simulink model "HANcoder_E407_Membership"  (R2022a)
settings: Solver=FixedStepDiscrete  StartTime=0.0  StopTime=1  FixedStep=0.01  RelTol=1e-3
PreLoadFcn:
  | librarySetup
  | eval([bdroot,'_startup']) %Calling [modelName]_startup.m
values from neighbouring files (symbols this model uses):
  HANtuneOverride = Simulink.Parameter    [HANcoder_E407_KinematicAngleControl_startup.m]    (also in HANcoder_E407_startup.m)
libraries: HANcoder_STM32_Target x14, simulink x2, simulink_extras x2, dspswit3 x1
settings Model: Creator=Jason van Kolfschoten  LastModifiedBy=luukr
settings SolverCC: AlgebraicLoopSolver=TrustRegion  PositivePriorityOrder=on
settings DataIOCC: LimitDataPoints=on  SaveFormat=Array  SignalLoggingSaveFormat=ModelDataLogs  SaveOutput=off  SignalLogging=off  DSMLogging=off  SaveTime=off  ReturnWorkspaceOutputs=off
settings OptimizationCC: BlockReduction=off  DefaultParameterBehavior=Inlined  DefaultUnderspecifiedDataType=single  InlineInvariantSignals=on  ExpressionDepthLimit=2147483647  StateBitsets=on  DataBitsets=on  ZeroExternalMemoryAtStartup=off  ZeroInternalMemoryAtStartup=off  InitFltsAndDblsToZero=on  NoFixptDivByZeroProtection=on  EfficientFloat2IntCast=on  LifeSpan=inf  EfficientTunableParamExpr=on
settings DebuggingCC: SaveWithDisabledLinksMsg=none  SaveWithParameterizedLinksMsg=none  CheckSSInitialOutputMsg=off  UnderspecifiedInitializationDetection=Classic  MergeDetectMultiDrivingBlocksExec=none  SignalResolutionControl=TryResolveAll  SolverPrmCheckMsg=warning  InheritedTsInSrcMsg=none  MultiTaskDSMMsg=warning  MultiTaskCondExecSysMsg=none  ParameterPrecisionLossMsg=none  FcnCallInpInsideContextMsg=warning  UnconnectedInputMsg=warning  UnconnectedOutputMsg=warning  UnconnectedLineMsg=warning  StateNameClashWarn=warning  SFUnexpectedBacktrackingDiag=warning  SFNoUnconditionalDefaultTransitionDiag=warning  SFExecutionAtInitializationDiag=none  SFMachineParentedDataDiag=warning  ArithmeticOperatorsInVariantConditions=warning
settings HardwareCC: ProdBitPerPointer=32  ProdBitPerSizeT=32  ProdBitPerPtrDiffT=32  ProdLargestAtomicInteger=Long  ProdLargestAtomicFloat=Double  ProdWordSize=32  ProdHWDeviceType=ARM Compatible->ARM Cortex  TargetEndianess=LittleEndian  TargetHWDeviceType=Infineon->TriCore
settings ModelReferenceCC: PropagateSignalLabelsOutOfModel=off
settings SFSimCC: SimUseLocalCustomCode=off  MATLABDynamicMemAlloc=off  CustomCodeUndefinedFunction=UseInterfaceOnly
settings RTWCC: Description=Real-Time Workshop Embedded Coder (no auto configuration)  SystemTargetFile=ert.tlc  MakeCommand=make_rtw SHELL= HANcoder_PORTABLE=1 HANcoder_BOOTLOADER=1  TemplateMakefile=STM32_E407_gcc.tmf  RTWUseLocalCustomCode=off
settings CodeAppCC: ForceParamTrailComments=on  IgnoreCustomStorageClasses=off  SimulinkDataObjDesc=on  CustomSymbolStrGlobalVar=rt$N$M  CustomSymbolStrType=$N$M  CustomSymbolStrFcn=$N$M$F  CustomSymbolStrMacro=$N$M  InsertBlockDesc=on  StateflowObjectComments=on  InternalIdentifier=Classic
settings ERTTargetCC: TargetFcnLib=ansi_tfl_tmw.mat  MultiwordLength=2048  IncludeMdlTerminateFcn=off  SuppressErrorStatus=on  SupportNonFinite=off  GenerateASAP2=on  InlinedParameterPlacement=NonHierarchical  ERTCustomFileTemplate=example_file_process.tlc  ConvertIfToSwitch=off  SuppressUnreachableDefaultCases=off
settings ConfigComp: CovMetricSettings=dw  CovSaveCumulativeToWorkspaceVar=on  CovSaveSingleToWorkspaceVar=on  CovExternalEMLEnable=off  CovSFcnEnable=off  DVMaxProcessTime=600  DVAutomaticStubbing=off  DVModelCoverageObjectives=MCDC  DVMaxTestCaseSteps=500  DVTestSuiteOptimization=CombinedObjectives  DVDetectActiveLogic=on  DVSaveHarnessModel=on  DVHarnessSource=Signal Editor

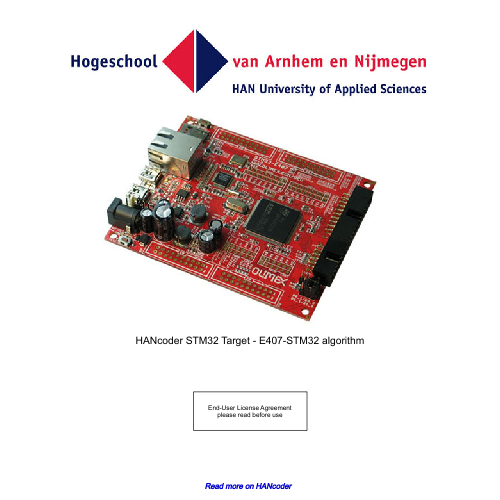
[thumbnail: Simulink's stored preview of the top-level diagram]
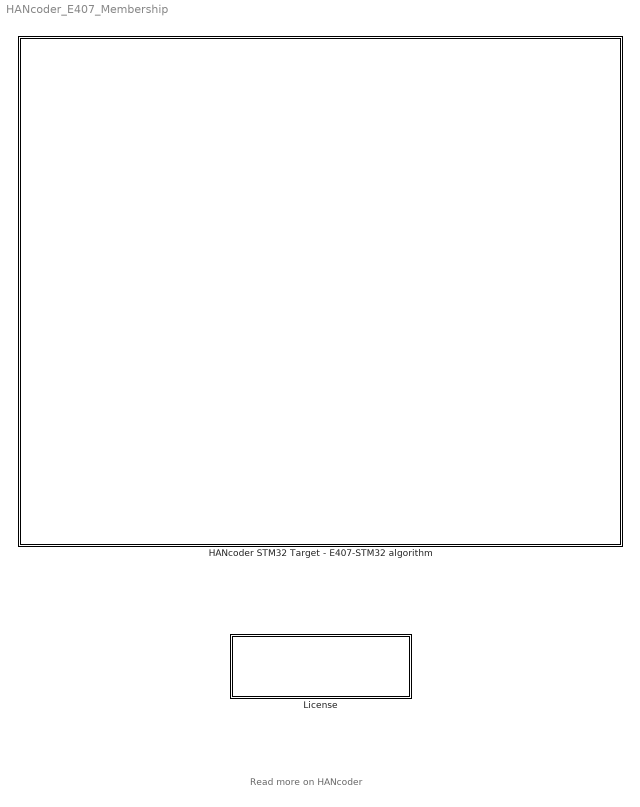
== system HANcoder_E407_Membership ==
  note: Read more on HANcoder
  HANcoder STM32 Target - E407-STM32 algorithm : Subsystem  mask(TopLevelSubsystem){}
      settings: CopyFcn=HANcoderChecks('Copy');  NameChangeFcn=HANcoderChecks('NameChangeE407');  MoveFcn=HANcoderChecks('MoveE407');
      mask Display: image(imread('STM32_E407_HAN.jpg'))
  License : Subsystem  mask(License){}
      settings: NameChangeFcn=HANcoderChecks('NameChangeLicenseBlock');  OpenFcn=winopen('License.pdf')  MoveFcn=HANcoderChecks('MoveLicenseBlock');
      mask Display: disp(['End-User License Agreement\n','please read before use']);

== system HANcoder_E407_Membership/HANcoder STM32 Target - E407-STM32 algorithm ==
  note: Template model
  Algorithm : Subsystem
  Base Sample Time config : HANcoder_STM32_Target/STM32-E407/System Config/Base Sample Time config  Tag=HANcoder_TARGET_STM32_E407  Description=HANcoder Target STM32-E407 blockset version 1.0  baseSampleTime=10  extraStack=100
      settings: SourceProductName=HANcoder STM32 Target
  Build settings : HANcoder_STM32_Target/STM32-E407/System Config/Build settings  Tag=HANcoder_TARGET_STM32_E407  AutoASAP2add=on  AutoFlash=USB
      settings: SourceProductName=HANcoder STM32 Target
  Custom ID config : HANcoder_STM32_Target/STM32-E407/System Config/Custom ID config  Tag=HANcoder_TARGET_STM32_E407  softID=softwareID  softNUM=1
      settings: SourceProductName=HANcoder STM32 Target
  Inputs : Subsystem
  Outputs : Subsystem
  Subsystem : Subsystem
  System information : Subsystem
  XCP on USB config : HANcoder_STM32_Target/STM32-E407/System Config/XCP on USB config  Tag=HANcoder_TARGET_STM32_E407
      settings: SourceProductName=HANcoder STM32 Target
  wires:
  Inputs/1(Button) -> Algorithm/1(Button)
  Algorithm/1(LED) -> Outputs/1(LED)

== system HANcoder_E407_Membership/License ==

== system HANcoder_E407_Membership/HANcoder STM32 Target - E407-STM32 algorithm/Algorithm ==
  note: The button or the HANtuneOverride parameter
      | switches between the two frequencies.
  note: Here the algorithm can be placed. No hardware dependent blocks should be used here.
  note: Switch LED frequency when button is pressed
  Button : Inport
  10Hz Counter Limiter : simulink/Sources/Counter Limited  uplimit=1  tsamp=0.1
  5Hz Counter Limited : simulink/Sources/Counter Limited  uplimit=1  tsamp=0.2
  Constant : Constant  Value=HANtuneOverride  OutDataTypeStr=boolean
  Data Type Conversion : DataTypeConversion  OutDataTypeStr=boolean  SaturateOnIntegerOverflow=off  RndMeth=Floor
  Logical Operator : Logic  Operator=OR  AllPortsSameDT=off  OutDataTypeStr=boolean
  Switch : Switch  Criteria=u2 > Threshold  SaturateOnIntegerOverflow=off  InputSameDT=off
  LED : Outport
  wires:
  Data Type Conversion/1 -> LED/1  "LedValue"
  5Hz Counter Limited/1 -> Switch/3
  Switch/1 -> Data Type Conversion/1
  Button/1 -> Logical Operator/2
  Logical Operator/1 -> Switch/2
  Constant/1 -> Logical Operator/1
  10Hz Counter Limiter/1 -> Switch/1

== system HANcoder_E407_Membership/HANcoder STM32 Target - E407-STM32 algorithm/Inputs ==
  note: The inputs and outputs are kept in a separate subsystem, this way the algorithm can easily be transferred to different hardware
  Digital Input : HANcoder_STM32_Target/STM32-E407/Digital Inputs/Digital Input  Tag=HANcoder_TARGET_STM32_E407  pinID=WKUP button  config=Pulldown  tsamp=-1
      settings: SourceProductName=HANcoder STM32 Target
  Button : Outport
  wires:
  Digital Input/1 -> Button/1

== system HANcoder_E407_Membership/HANcoder STM32 Target - E407-STM32 algorithm/Outputs ==
  note: The inputs and outputs are kept in a separate subsystem, this way the algorithm can easily be transferred to different hardware
  LED : Inport
  Digital Output : HANcoder_STM32_Target/STM32-E407/Digital Outputs/Digital Output  Tag=HANcoder_TARGET_STM32_E407  pinID=LED  config=Push pull  tsamp=-1
      settings: SourceProductName=HANcoder STM32 Target
  wires:
  LED/1 -> Digital Output/1

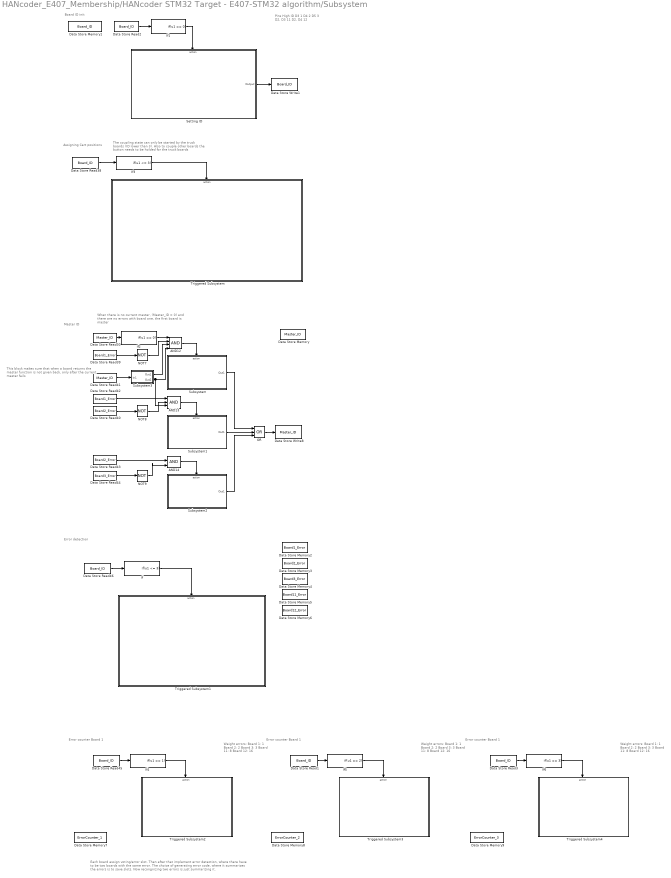
== system HANcoder_E407_Membership/HANcoder STM32 Target - E407-STM32 algorithm/Subsystem ==
  note: Each board assign voting/error slot. Then after that implement error detection, where there have to be two boards with the same error. The choice of generating error code, where it summarizes the errors is to save slots. Now recongnizing two errors is just summarizing it.
  note: Weight errors:
      | Board 1: 1
      | Board 2: 2
      | Board 3: 3
      | Board 11: 8
      | Board 12: 16
  note: Error counter Board 1
  note: Error detection
  note: Assigning Cart positions
  note: This block makes sure that when a board returns the master function is not given back, only after the current master fails
  note: Master ID
  note: Board ID init
  note: Pins High      		ID
      | D3                 		1
      | D4				2
      | D5				3
      | D2, D3			11
      | D2, D4			12
  note: When there is no current master, (Master_ID = 0) and there are no errors with board one, the first board is master
  note: The coupling state can only be started by the truck boards (ID lower than 3). Also to couple other boards the button needs to be holded for the truck boards
  note: Weight errors:
      | Board 1: 1
      | Board 2: 2
      | Board 3: 3
      | Board 11: 8
      | Board 12: 16
  note: Error counter Board 1
  note: Weight errors:
      | Board 1: 1
      | Board 2: 2
      | Board 3: 3
      | Board 11: 8
      | Board 12: 16
  note: Error counter Board 1
  AND12 : Logic  Inputs=4  IconShape=distinctive  AllPortsSameDT=off  OutDataTypeStr=boolean
  AND13 : Logic  Inputs=3  IconShape=distinctive  AllPortsSameDT=off  OutDataTypeStr=boolean
  AND14 : Logic  IconShape=distinctive  AllPortsSameDT=off  OutDataTypeStr=boolean
  Data Store Memory : DataStoreMemory  DataStoreName=Master_ID  WriteAfterWriteMsg=warning  ShowAdditionalParam=off
  Data Store Memory1 : DataStoreMemory  Priority=10  DataStoreName=Board_ID  ReadBeforeWriteMsg=warning  WriteAfterWriteMsg=warning  WriteAfterReadMsg=warning  ShowAdditionalParam=off
  Data Store Memory2 : DataStoreMemory  DataStoreName=Board1_Error  WriteAfterWriteMsg=warning  ShowAdditionalParam=off
  Data Store Memory3 : DataStoreMemory  DataStoreName=Board2_Error  WriteAfterWriteMsg=warning  ShowAdditionalParam=off
  Data Store Memory4 : DataStoreMemory  DataStoreName=Board3_Error  WriteAfterWriteMsg=warning  ShowAdditionalParam=off
  Data Store Memory5 : DataStoreMemory  DataStoreName=Board11_Error  WriteAfterWriteMsg=warning  ShowAdditionalParam=off
  Data Store Memory6 : DataStoreMemory  DataStoreName=Board12_Error  WriteAfterWriteMsg=warning  ShowAdditionalParam=off
  Data Store Memory7 : DataStoreMemory  DataStoreName=ErrorCounter_1  WriteAfterWriteMsg=warning  ShowAdditionalParam=off
  Data Store Memory8 : DataStoreMemory  DataStoreName=ErrorCounter_2  WriteAfterWriteMsg=warning  ShowAdditionalParam=off
  Data Store Memory9 : DataStoreMemory  DataStoreName=ErrorCounter_3  WriteAfterWriteMsg=warning  ShowAdditionalParam=off
  Data Store Read{1,3,38,45..46} (5 alike) : DataStoreRead  DataStoreName=Board_ID  IndexOptions=Index vector (dialog)  Indices=1  OutputSizes=1
  Data Store Read2 : DataStoreRead  Priority=10  DataStoreName=Board_ID  IndexOptions=Index vector (dialog)  Indices=1  OutputSizes=1
  Data Store Read30 : DataStoreRead  DataStoreName=Master_ID  IndexOptions=Index vector (dialog)  Indices=1  OutputSizes=1
  Data Store Read39 : DataStoreRead  DataStoreName=Board1_Error  IndexOptions=Index vector (dialog)  Indices=1  OutputSizes=1
  Data Store Read40 : DataStoreRead  DataStoreName=Board2_Error  IndexOptions=Index vector (dialog)  Indices=1  OutputSizes=1
  Data Store Read41 : DataStoreRead  DataStoreName=Master_ID  IndexOptions=Index vector (dialog)  Indices=1  OutputSizes=1
  Data Store Read42 : DataStoreRead  DataStoreName=Board1_Error  IndexOptions=Index vector (dialog)  Indices=1  OutputSizes=1
  Data Store Read43 : DataStoreRead  DataStoreName=Board2_Error  IndexOptions=Index vector (dialog)  Indices=1  OutputSizes=1
  Data Store Read44 : DataStoreRead  DataStoreName=Board3_Error  IndexOptions=Index vector (dialog)  Indices=1  OutputSizes=1
  Data Store Write1 : DataStoreWrite  Priority=13  DataStoreName=Board_ID  IndexOptions=Index vector (dialog)  Indices=1  OutputSizes=1
  Data Store Write8 : DataStoreWrite  Priority=13  DataStoreName=Master_ID  IndexOptions=Index vector (dialog)  Indices=1  OutputSizes=1
  If : If  IfExpression=u1 <= 3  ShowElse=off
  If1 : If  Priority=11  IfExpression=u1 == 0  ShowElse=off
  If2 : If  Priority=11  IfExpression=u1 == 0  ShowElse=off
  If3 : If  Priority=11  IfExpression=u1 <= 3  ShowElse=off
  If4 : If  IfExpression=u1 == 1  ShowElse=off
  If5 : If  IfExpression=u1 == 2  ShowElse=off
  If6 : If  IfExpression=u1 == 3  ShowElse=off
  NOT7 : Logic  Operator=NOT  IconShape=distinctive  AllPortsSameDT=off  OutDataTypeStr=boolean
  NOT8 : Logic  Operator=NOT  IconShape=distinctive  AllPortsSameDT=off  OutDataTypeStr=boolean
  NOT9 : Logic  Operator=NOT  IconShape=distinctive  AllPortsSameDT=off  OutDataTypeStr=boolean
  OR : Logic  Operator=OR  Inputs=3  IconShape=distinctive  AllPortsSameDT=off  OutDataTypeStr=boolean
  Setting ID : Subsystem
  Subsystem : Subsystem
  Subsystem1 : Subsystem
  Subsystem2 : Subsystem
  Subsystem3 : Subsystem
  Triggered Subsystem : Subsystem  TreatAsAtomicUnit=on
  Triggered Subsystem1 : Subsystem  TreatAsAtomicUnit=on
  Triggered Subsystem2 : Subsystem  TreatAsAtomicUnit=on
  Triggered Subsystem3 : Subsystem  TreatAsAtomicUnit=on
  Triggered Subsystem4 : Subsystem  TreatAsAtomicUnit=on
  wires:
  If1/1 -> Setting ID/Action
  Data Store Read2/1 -> If1/1
  Setting ID/1(Output) -> Data Store Write1/1
  Data Store Read30/1 -> If2/1
  Data Store Read38/1 -> If3/1
  OR/1 -> Data Store Write8/1
  Subsystem1/1(Out1) -> OR/2
  Subsystem/1(Out1) -> OR/1
  Subsystem2/1(Out1) -> OR/3
  Data Store Read39/1 -> NOT7/1
  If2/1 -> AND12/1
  AND12/1 -> Subsystem/Action
  NOT7/1 -> AND12/2
  NOT8/1 -> AND13/2
  Data Store Read40/1 -> NOT8/1
  Data Store Read42/1 -> AND13/1
  AND13/1 -> Subsystem1/Action
  Data Store Read44/1 -> NOT9/1
  NOT9/1 -> AND14/2
  Data Store Read43/1 -> AND14/1
  AND14/1 -> Subsystem2/Action
  Data Store Read41/1 -> Subsystem3/1(In1)
  Subsystem3/1(Out1) -> AND12/3
  Subsystem3/2(Out2) -> AND13/3, AND12/4
  If3/1 -> Triggered Subsystem/Action
  Data Store Read45/1 -> If4/1
  Data Store Read46/1 -> If/1
  If/1 -> Triggered Subsystem1/Action
  If4/1 -> Triggered Subsystem2/Action
  If5/1 -> Triggered Subsystem3/Action
  Data Store Read1/1 -> If5/1
  Data Store Read3/1 -> If6/1
  If6/1 -> Triggered Subsystem4/Action

== system HANcoder_E407_Membership/HANcoder STM32 Target - E407-STM32 algorithm/System information ==
  note: These blocks check the free memory: stack and heap and the CPU load,
      | this way you can see whether your software demands too much of the microcontroller
  Get CPU load : HANcoder_STM32_Target/STM32-E407/System Management/Get CPU load  Tag=HANcoder_TARGET_STM32_E407  mode=Current CPU load  tsamp=-1
      settings: SourceProductName=HANcoder STM32 Target
  Get free Heap : HANcoder_STM32_Target/STM32-E407/System Management/Get free Heap  Tag=HANcoder_TARGET_STM32_E407  tsamp=-1
      settings: SourceProductName=HANcoder STM32 Target
  Get free Stack : HANcoder_STM32_Target/STM32-E407/System Management/Get free Stack  Tag=HANcoder_TARGET_STM32_E407  taskIdx=Application Control Task  tsamp=-1
      settings: SourceProductName=HANcoder STM32 Target
  Terminator : Terminator
  Terminator1 : Terminator
  Terminator2 : Terminator
  wires:
  Get CPU load/1 -> Terminator1/1  "SI_CPUload"
  Get free Stack/1 -> Terminator/1  "SI_FreeStack"
  Get free Heap/1 -> Terminator2/1  "SI_FreeHeap"

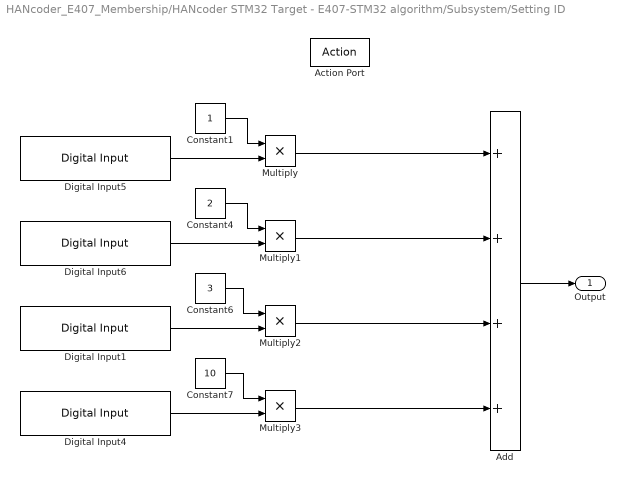
== system HANcoder_E407_Membership/HANcoder STM32 Target - E407-STM32 algorithm/Subsystem/Setting ID ==
  Action Port : ActionPort  ActionPortLabel=if(u1 == 0)
  Add : Sum  Inputs=++++
  Constant1 : Constant
  Constant4 : Constant  Value=2
  Constant6 : Constant  Value=3
  Constant7 : Constant  Value=10
  Digital Input1 : HANcoder_STM32_Target/STM32-E407/Digital Inputs/Digital Input  Tag=HANcoder_TARGET_STM32_E407  pinID=CON3 - D5 - 5V Tolerant  config=Pulldown  tsamp=-1
      settings: SourceProductName=HANcoder STM32 Target
  Digital Input4 : HANcoder_STM32_Target/STM32-E407/Digital Inputs/Digital Input  Tag=HANcoder_TARGET_STM32_E407  pinID=CON3 - D2 - 5V Tolerant  config=Pulldown  tsamp=-1
      settings: SourceProductName=HANcoder STM32 Target
  Digital Input5 : HANcoder_STM32_Target/STM32-E407/Digital Inputs/Digital Input  Tag=HANcoder_TARGET_STM32_E407  pinID=CON3 - D3 - 5V Tolerant  config=Pulldown  tsamp=-1
      settings: SourceProductName=HANcoder STM32 Target
  Digital Input6 : HANcoder_STM32_Target/STM32-E407/Digital Inputs/Digital Input  Tag=HANcoder_TARGET_STM32_E407  pinID=CON3 - D4 - 5V Tolerant  config=Pulldown  tsamp=-1
      settings: SourceProductName=HANcoder STM32 Target
  Multiply{,1..3} (4 alike) : Product
  Output : Outport
  wires:
  Constant4/1 -> Multiply1/1
  Multiply/1 -> Add/1
  Constant1/1 -> Multiply/1
  Multiply1/1 -> Add/2
  Multiply2/1 -> Add/3
  Constant6/1 -> Multiply2/1
  Digital Input5/1 -> Multiply/2
  Digital Input6/1 -> Multiply1/2
  Digital Input1/1 -> Multiply2/2
  Constant7/1 -> Multiply3/1
  Multiply3/1 -> Add/4
  Digital Input4/1 -> Multiply3/2
  Add/1 -> Output/1

== system HANcoder_E407_Membership/HANcoder STM32 Target - E407-STM32 algorithm/Subsystem/Subsystem ==
  Action Port : ActionPort
  Constant : Constant
  Data Store Read1 : DataStoreRead  Priority=10  DataStoreName=Board_ID  IndexOptions=Index vector (dialog)  Indices=1  OutputSizes=1
  Equal1 : RelationalOperator  Operator===  OutDataTypeStr=boolean  RndMeth=Simplest  InputSameDT=off
  Out1 : Outport
  wires:
  Constant/1 -> Equal1/2
  Equal1/1 -> Out1/1
  Data Store Read1/1 -> Equal1/1

== system HANcoder_E407_Membership/HANcoder STM32 Target - E407-STM32 algorithm/Subsystem/Subsystem1 ==
  Action Port : ActionPort
  Constant : Constant  Value=2
  Data Store Read1 : DataStoreRead  Priority=10  DataStoreName=Board_ID  IndexOptions=Index vector (dialog)  Indices=1  OutputSizes=1
  Equal1 : RelationalOperator  Operator===  OutDataTypeStr=boolean  RndMeth=Simplest  InputSameDT=off
  Out1 : Outport
  wires:
  Data Store Read1/1 -> Equal1/1
  Equal1/1 -> Out1/1
  Constant/1 -> Equal1/2

== system HANcoder_E407_Membership/HANcoder STM32 Target - E407-STM32 algorithm/Subsystem/Subsystem2 ==
  Action Port : ActionPort
  Constant : Constant  Value=3
  Data Store Read1 : DataStoreRead  Priority=10  DataStoreName=Board_ID  IndexOptions=Index vector (dialog)  Indices=1  OutputSizes=1
  Equal1 : RelationalOperator  Operator===  OutDataTypeStr=boolean  RndMeth=Simplest  InputSameDT=off
  Out1 : Outport
  wires:
  Constant/1 -> Equal1/2
  Equal1/1 -> Out1/1
  Data Store Read1/1 -> Equal1/1

== system HANcoder_E407_Membership/HANcoder STM32 Target - E407-STM32 algorithm/Subsystem/Subsystem3 ==
  In1 : Inport
  If : If  IfExpression=u1 == 2  ShowElse=off
  If4 : If  IfExpression=u1 == 3  ShowElse=off
  NOT10 : Logic  Operator=NOT  IconShape=distinctive  AllPortsSameDT=off  OutDataTypeStr=boolean
  NOT11 : Logic  Operator=NOT  IconShape=distinctive  AllPortsSameDT=off  OutDataTypeStr=boolean
  Out1 : Outport
  Out2 : Outport  Port=2
  wires:
  NOT11/1 -> Out2/1
  In1/1 -> If4/1, If/1
  If/1 -> NOT10/1
  If4/1 -> NOT11/1
  NOT10/1 -> Out1/1

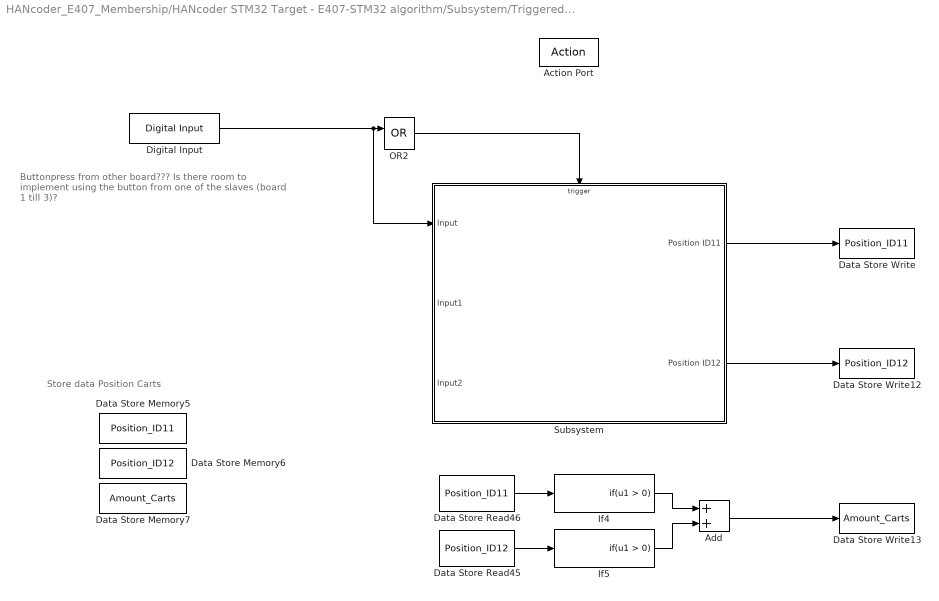
== system HANcoder_E407_Membership/HANcoder STM32 Target - E407-STM32 algorithm/Subsystem/Triggered Subsystem ==
  note: Store data Position Carts
  note: Buttonpress from other board??? Is there room to implement using the button from one of the slaves (board 1 till 3)?
  Action Port : ActionPort  ActionPortLabel=if(u1 <= 3)
  Add : Sum
  Data Store Memory5 : DataStoreMemory  DataStoreName=Position_ID11  WriteAfterWriteMsg=warning  ShowAdditionalParam=off
  Data Store Memory6 : DataStoreMemory  DataStoreName=Position_ID12  WriteAfterWriteMsg=warning  ShowAdditionalParam=off
  Data Store Memory7 : DataStoreMemory  DataStoreName=Amount_Carts  WriteAfterWriteMsg=warning  ShowAdditionalParam=off
  Data Store Read45 : DataStoreRead  DataStoreName=Position_ID12  IndexOptions=Index vector (dialog)  Indices=1  OutputSizes=1
  Data Store Read46 : DataStoreRead  DataStoreName=Position_ID11  IndexOptions=Index vector (dialog)  Indices=1  OutputSizes=1
  Data Store Write : DataStoreWrite  DataStoreName=Position_ID11  IndexOptions=Index vector (dialog)  Indices=1  OutputSizes=1
  Data Store Write12 : DataStoreWrite  DataStoreName=Position_ID12  IndexOptions=Index vector (dialog)  Indices=1  OutputSizes=1
  Data Store Write13 : DataStoreWrite  DataStoreName=Amount_Carts  IndexOptions=Index vector (dialog)  Indices=1  OutputSizes=1
  Digital Input : HANcoder_STM32_Target/STM32-E407/Digital Inputs/Digital Input  Tag=HANcoder_TARGET_STM32_E407  pinID=WKUP button  config=Pulldown  tsamp=-1
      settings: SourceProductName=HANcoder STM32 Target
  If4 : If  ShowElse=off
  If5 : If  ShowElse=off
  OR2 : Logic  Operator=OR  IconShape=distinctive  AllPortsSameDT=off  OutDataTypeStr=boolean
  Subsystem : Subsystem
  wires:
  Digital Input/1 -> Subsystem/1(Input), OR2/1
  ? -> OR2/2
  OR2/1 -> Subsystem/Trigger
  Add/1 -> Data Store Write13/1
  Subsystem/1(Position ID11) -> Data Store Write/1
  Subsystem/2(Position ID12) -> Data Store Write12/1
  Data Store Read45/1 -> If5/1
  If5/1 -> Add/2
  If4/1 -> Add/1
  Data Store Read46/1 -> If4/1

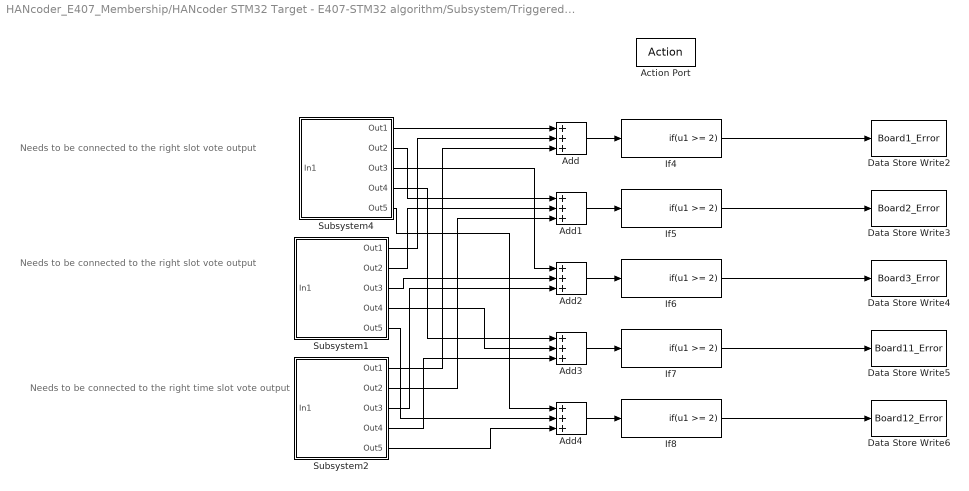
== system HANcoder_E407_Membership/HANcoder STM32 Target - E407-STM32 algorithm/Subsystem/Triggered Subsystem1 ==
  note: Needs to be connected to the right slot vote output
  note: Needs to be connected to the right slot vote output
  note: Needs to be connected to the right time slot vote output
  Action Port : ActionPort  ActionPortLabel=if(u1 <= 3)
  Add{,1..4} (5 alike) : Sum  Inputs=+++
  Data Store Write2 : DataStoreWrite  Priority=13  DataStoreName=Board1_Error  IndexOptions=Index vector (dialog)  Indices=1  OutputSizes=1
  Data Store Write3 : DataStoreWrite  Priority=13  DataStoreName=Board2_Error  IndexOptions=Index vector (dialog)  Indices=1  OutputSizes=1
  Data Store Write4 : DataStoreWrite  Priority=13  DataStoreName=Board3_Error  IndexOptions=Index vector (dialog)  Indices=1  OutputSizes=1
  Data Store Write5 : DataStoreWrite  Priority=13  DataStoreName=Board11_Error  IndexOptions=Index vector (dialog)  Indices=1  OutputSizes=1
  Data Store Write6 : DataStoreWrite  Priority=13  DataStoreName=Board12_Error  IndexOptions=Index vector (dialog)  Indices=1  OutputSizes=1
  If{4..8} (5 alike) : If  IfExpression=u1 >= 2  ShowElse=off
  Subsystem1 : Subsystem
  Subsystem2 : Subsystem
  Subsystem4 : Subsystem
  wires:
  If4/1 -> Data Store Write2/1
  Add1/1 -> If5/1
  Subsystem1/5(Out5) -> Add4/2
  Subsystem2/4(Out4) -> Add3/3
  Add/1 -> If4/1
  Add2/1 -> If6/1
  Add3/1 -> If7/1
  Subsystem1/2(Out2) -> Add1/2
  Subsystem2/5(Out5) -> Add4/3
  Subsystem4/1(Out1) -> Add/1
  If5/1 -> Data Store Write3/1
  If6/1 -> Data Store Write4/1
  Subsystem4/4(Out4) -> Add3/1
  If8/1 -> Data Store Write6/1
  Subsystem4/5(Out5) -> Add4/1
  Add4/1 -> If8/1
  Subsystem2/1(Out1) -> Add/3
  Subsystem1/4(Out4) -> Add3/2
  Subsystem2/3(Out3) -> Add2/3
  Subsystem1/1(Out1) -> Add/2
  Subsystem4/3(Out3) -> Add2/1
  If7/1 -> Data Store Write5/1
  Subsystem2/2(Out2) -> Add1/3
  Subsystem4/2(Out2) -> Add1/1
  Subsystem1/3(Out3) -> Add2/2
  ? -> Subsystem4/1(In1)
  ? -> Subsystem1/1(In1)
  ? -> Subsystem2/1(In1)

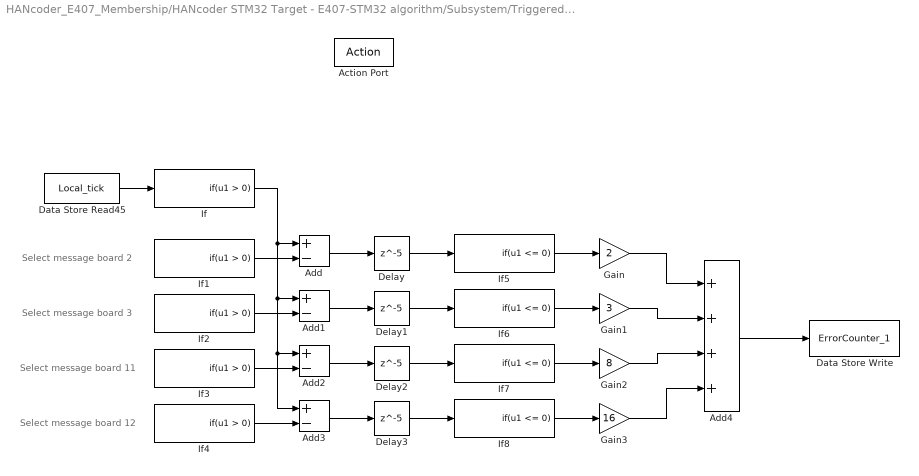
== system HANcoder_E407_Membership/HANcoder STM32 Target - E407-STM32 algorithm/Subsystem/Triggered Subsystem2 ==
  note: Select message board 2
  note: Select message board 3
  note: Select message board 11
  note: Select message board 12
  Action Port : ActionPort  ActionPortLabel=if(u1 == 1)
  Add{,1..3} (4 alike) : Sum  Inputs=+-
  Add4 : Sum  Inputs=++++
  Data Store Read45 : DataStoreRead  DataStoreName=Local_tick  IndexOptions=Index vector (dialog)  Indices=1  OutputSizes=1
  Data Store Write : DataStoreWrite  DataStoreName=ErrorCounter_1  IndexOptions=Index vector (dialog)  Indices=1  OutputSizes=1
  Delay{,1..3} (4 alike) : Delay  DelayLength=5
  Gain : Gain  Gain=2
  Gain1 : Gain  Gain=3
  Gain2 : Gain  Gain=8
  Gain3 : Gain  Gain=16
  If{,1..4} (5 alike) : If  ShowElse=off
  If{5..8} (4 alike) : If  IfExpression=u1 <= 0  ShowElse=off
  wires:
  Data Store Read45/1 -> If/1
  If1/1 -> Add/2
  Add/1 -> Delay/1
  If2/1 -> Add1/2
  If3/1 -> Add2/2
  If/1 -> Add3/1, Add2/1, Add1/1, Add/1
  If4/1 -> Add3/2
  Add1/1 -> Delay1/1
  Add2/1 -> Delay2/1
  Add3/1 -> Delay3/1
  Delay/1 -> If5/1
  Delay1/1 -> If6/1
  Delay2/1 -> If7/1
  Delay3/1 -> If8/1
  If8/1 -> Gain3/1
  If7/1 -> Gain2/1
  If6/1 -> Gain1/1
  If5/1 -> Gain/1
  Gain/1 -> Add4/1
  Gain1/1 -> Add4/2
  Gain2/1 -> Add4/3
  Gain3/1 -> Add4/4
  Add4/1 -> Data Store Write/1

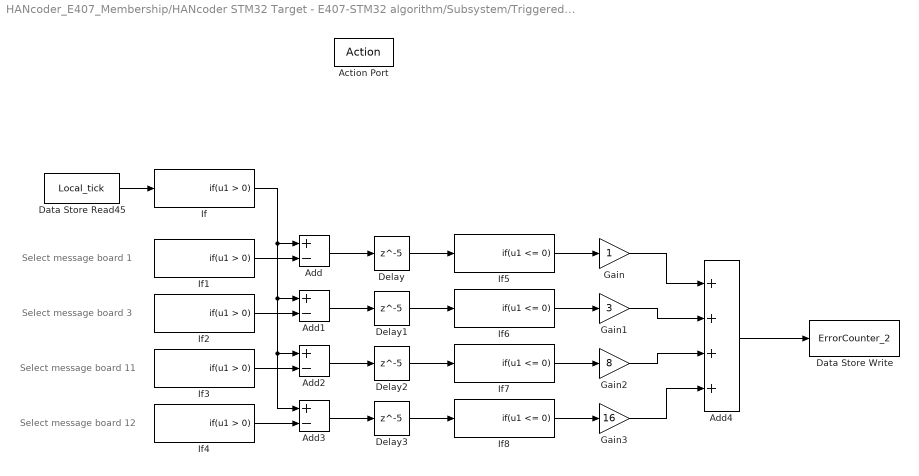
== system HANcoder_E407_Membership/HANcoder STM32 Target - E407-STM32 algorithm/Subsystem/Triggered Subsystem3 ==
  note: Select message board 12
  note: Select message board 11
  note: Select message board 3
  note: Select message board 1
  Action Port : ActionPort  ActionPortLabel=if(u1 == 1)
  Add{,1..3} (4 alike) : Sum  Inputs=+-
  Add4 : Sum  Inputs=++++
  Data Store Read45 : DataStoreRead  DataStoreName=Local_tick  IndexOptions=Index vector (dialog)  Indices=1  OutputSizes=1
  Data Store Write : DataStoreWrite  DataStoreName=ErrorCounter_2  IndexOptions=Index vector (dialog)  Indices=1  OutputSizes=1
  Delay{,1..3} (4 alike) : Delay  DelayLength=5
  Gain : Gain
  Gain1 : Gain  Gain=3
  Gain2 : Gain  Gain=8
  Gain3 : Gain  Gain=16
  If{,1..4} (5 alike) : If  ShowElse=off
  If{5..8} (4 alike) : If  IfExpression=u1 <= 0  ShowElse=off
  wires:
  Add4/1 -> Data Store Write/1
  Gain3/1 -> Add4/4
  Gain2/1 -> Add4/3
  Gain1/1 -> Add4/2
  Gain/1 -> Add4/1
  If5/1 -> Gain/1
  If6/1 -> Gain1/1
  If7/1 -> Gain2/1
  If8/1 -> Gain3/1
  Delay3/1 -> If8/1
  Delay2/1 -> If7/1
  Delay1/1 -> If6/1
  Delay/1 -> If5/1
  Add3/1 -> Delay3/1
  Add2/1 -> Delay2/1
  Add1/1 -> Delay1/1
  If4/1 -> Add3/2
  If/1 -> Add/1, Add1/1, Add2/1, Add3/1
  If3/1 -> Add2/2
  If2/1 -> Add1/2
  Add/1 -> Delay/1
  If1/1 -> Add/2
  Data Store Read45/1 -> If/1

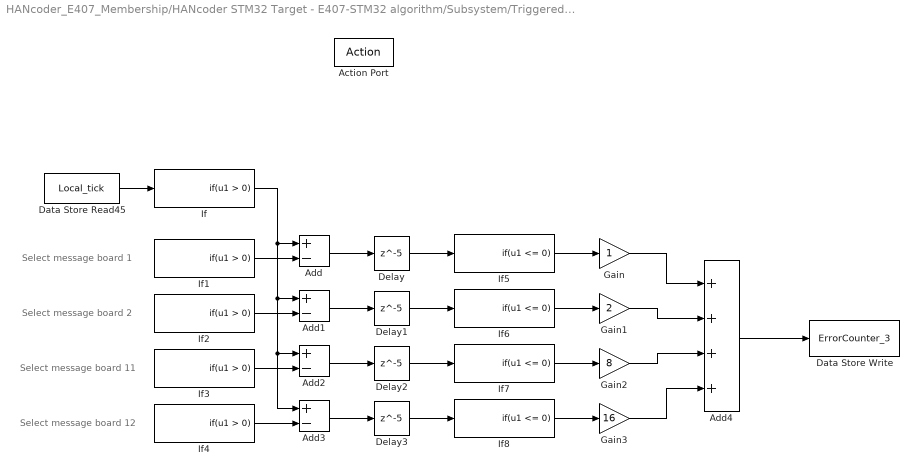
== system HANcoder_E407_Membership/HANcoder STM32 Target - E407-STM32 algorithm/Subsystem/Triggered Subsystem4 ==
  note: Select message board 1
  note: Select message board 2
  note: Select message board 11
  note: Select message board 12
  Action Port : ActionPort  ActionPortLabel=if(u1 == 2)
  Add{,1..3} (4 alike) : Sum  Inputs=+-
  Add4 : Sum  Inputs=++++
  Data Store Read45 : DataStoreRead  DataStoreName=Local_tick  IndexOptions=Index vector (dialog)  Indices=1  OutputSizes=1
  Data Store Write : DataStoreWrite  DataStoreName=ErrorCounter_3  IndexOptions=Index vector (dialog)  Indices=1  OutputSizes=1
  Delay{,1..3} (4 alike) : Delay  DelayLength=5
  Gain : Gain
  Gain1 : Gain  Gain=2
  Gain2 : Gain  Gain=8
  Gain3 : Gain  Gain=16
  If{,1..4} (5 alike) : If  ShowElse=off
  If{5..8} (4 alike) : If  IfExpression=u1 <= 0  ShowElse=off
  wires:
  Data Store Read45/1 -> If/1
  If1/1 -> Add/2
  Add/1 -> Delay/1
  If2/1 -> Add1/2
  If3/1 -> Add2/2
  If/1 -> Add3/1, Add2/1, Add1/1, Add/1
  If4/1 -> Add3/2
  Add1/1 -> Delay1/1
  Add2/1 -> Delay2/1
  Add3/1 -> Delay3/1
  Delay/1 -> If5/1
  Delay1/1 -> If6/1
  Delay2/1 -> If7/1
  Delay3/1 -> If8/1
  If8/1 -> Gain3/1
  If7/1 -> Gain2/1
  If6/1 -> Gain1/1
  If5/1 -> Gain/1
  Gain/1 -> Add4/1
  Gain1/1 -> Add4/2
  Gain2/1 -> Add4/3
  Gain3/1 -> Add4/4
  Add4/1 -> Data Store Write/1

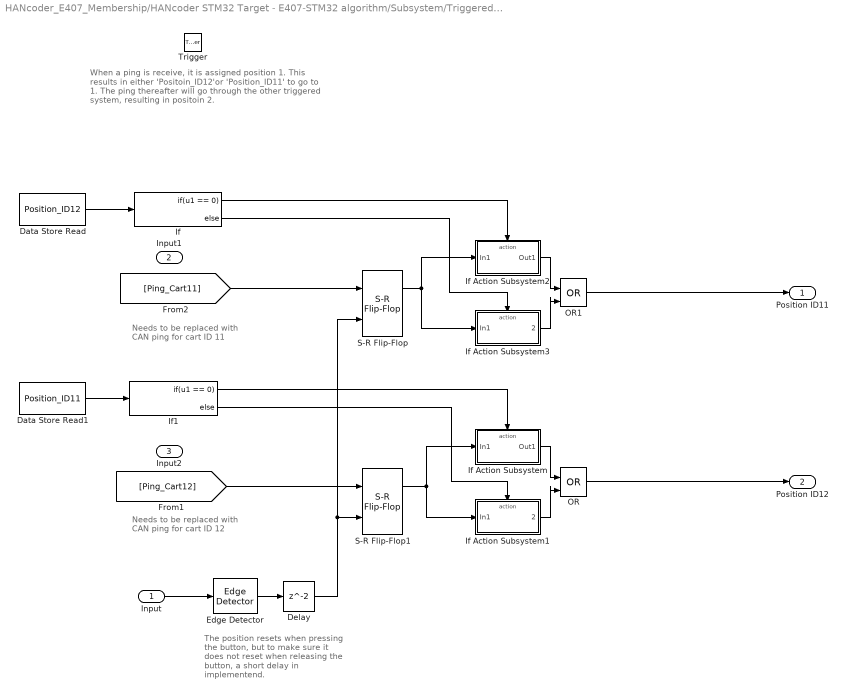
== system HANcoder_E407_Membership/HANcoder STM32 Target - E407-STM32 algorithm/Subsystem/Triggered Subsystem/Subsystem ==
  note: The position resets when pressing the button, but to make sure it does not reset when releasing the button, a short delay in implementend.
  note: When a ping is receive, it is assigned position 1. This results in either 'Positoin_ID12'or 'Position_ID11' to go to 1. The ping thereafter will go through the other triggered system, resulting in positoin 2.
  note: Needs to be replaced with CAN ping for cart ID 12
  note: Needs to be replaced with CAN ping for cart ID 11
  Input : Inport
  Input1 : Inport  Port=2
  Input2 : Inport  Port=3
  Trigger : TriggerPort  TriggerType=function-call  VariantControl=(inherit)  PortDimensions=1
  Data Store Read : DataStoreRead  DataStoreName=Position_ID12  IndexOptions=Index vector (dialog)  Indices=1  OutputSizes=1
  Data Store Read1 : DataStoreRead  DataStoreName=Position_ID11  IndexOptions=Index vector (dialog)  Indices=1  OutputSizes=1
  Delay : Delay
  Edge Detector : dspswit3/Edge Detector  InputProcessing=Columns as channels (frame based)
      settings: SourceProductBaseCode=DS
  If : If  IfExpression=u1 == 0
  If Action Subsystem : Subsystem  TreatAsAtomicUnit=on
  If Action Subsystem1 : Subsystem  TreatAsAtomicUnit=on
  If Action Subsystem2 : Subsystem  TreatAsAtomicUnit=on
  If Action Subsystem3 : Subsystem  TreatAsAtomicUnit=on
  If1 : If  IfExpression=u1 == 0
  OR : Logic  Operator=OR  IconShape=distinctive  AllPortsSameDT=off  OutDataTypeStr=boolean
  OR1 : Logic  Operator=OR  IconShape=distinctive  AllPortsSameDT=off  OutDataTypeStr=boolean
  S-R Flip-Flop : simulink_extras/Flip Flops/S-R Flip-Flop  initial_condition=0
  S-R Flip-Flop1 : simulink_extras/Flip Flops/S-R Flip-Flop  initial_condition=0
  Position ID11 : Outport
  Position ID12 : Outport  Port=2
  wires:
  Delay/1 -> S-R Flip-Flop/2, S-R Flip-Flop1/2
  Data Store Read1/1 -> If1/1
  If Action Subsystem3/1(2) -> OR1/2
  If Action Subsystem1/1(2) -> OR/2
  If Action Subsystem/1(Out1) -> OR/1
  S-R Flip-Flop1/1 -> If Action Subsystem/1(In1), If Action Subsystem1/1(In1)
  [Ping_Cart11] -> S-R Flip-Flop/1
  If Action Subsystem2/1(Out1) -> OR1/1
  If1/1 -> If Action Subsystem/Action
  S-R Flip-Flop/1 -> If Action Subsystem3/1(In1), If Action Subsystem2/1(In1)
  Input/1 -> Edge Detector/1
  Edge Detector/1 -> Delay/1
  OR/1 -> Position ID12/1
  If/2 -> If Action Subsystem3/Action
  [Ping_Cart12] -> S-R Flip-Flop1/1
  If/1 -> If Action Subsystem2/Action
  Data Store Read/1 -> If/1
  If1/2 -> If Action Subsystem1/Action
  OR1/1 -> Position ID11/1

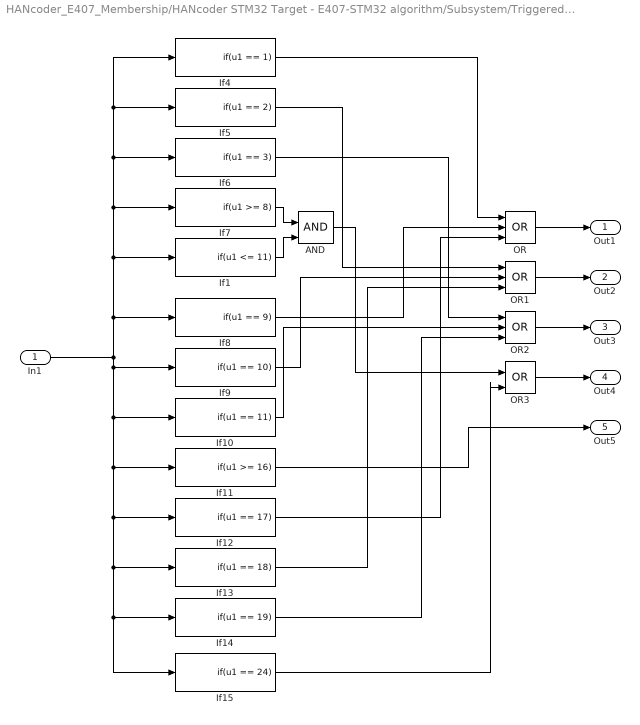
== system HANcoder_E407_Membership/HANcoder STM32 Target - E407-STM32 algorithm/Subsystem/Triggered Subsystem1/Subsystem1 ==
  In1 : Inport
  AND : Logic  IconShape=distinctive  AllPortsSameDT=off  OutDataTypeStr=boolean
  If1 : If  IfExpression=u1 <= 11  ShowElse=off
  If10 : If  IfExpression=u1 == 11  ShowElse=off
  If11 : If  IfExpression=u1 >= 16  ShowElse=off
  If12 : If  IfExpression=u1 == 17  ShowElse=off
  If13 : If  IfExpression=u1 == 18  ShowElse=off
  If14 : If  IfExpression=u1 == 19  ShowElse=off
  If15 : If  IfExpression=u1 == 24  ShowElse=off
  If4 : If  IfExpression=u1 == 1  ShowElse=off
  If5 : If  IfExpression=u1 == 2  ShowElse=off
  If6 : If  IfExpression=u1 == 3  ShowElse=off
  If7 : If  IfExpression=u1 >= 8  ShowElse=off
  If8 : If  IfExpression=u1 == 9  ShowElse=off
  If9 : If  IfExpression=u1 == 10  ShowElse=off
  OR : Logic  Operator=OR  Inputs=3  IconShape=distinctive  AllPortsSameDT=off  OutDataTypeStr=boolean
  OR1 : Logic  Operator=OR  Inputs=3  IconShape=distinctive  AllPortsSameDT=off  OutDataTypeStr=boolean
  OR2 : Logic  Operator=OR  Inputs=3  IconShape=distinctive  AllPortsSameDT=off  OutDataTypeStr=boolean
  OR3 : Logic  Operator=OR  IconShape=distinctive  AllPortsSameDT=off  OutDataTypeStr=boolean
  Out1 : Outport
  Out2 : Outport  Port=2
  Out3 : Outport  Port=3
  Out4 : Outport  Port=4
  Out5 : Outport  Port=5
  wires:
  AND/1 -> OR3/1
  If1/1 -> AND/2
  If7/1 -> AND/1
  If11/1 -> Out5/1
  OR3/1 -> Out4/1
  If15/1 -> OR3/2
  If14/1 -> OR2/3
  If10/1 -> OR2/2
  If6/1 -> OR2/1
  OR2/1 -> Out3/1
  If13/1 -> OR1/3
  If9/1 -> OR1/2
  If5/1 -> OR1/1
  OR1/1 -> Out2/1
  If12/1 -> OR/3
  If8/1 -> OR/2
  If4/1 -> OR/1
  OR/1 -> Out1/1
  In1/1 -> If8/1, If4/1, If5/1, If6/1, If7/1, If1/1, If9/1, If10/1, If11/1, If12/1, If15/1, If14/1, If13/1

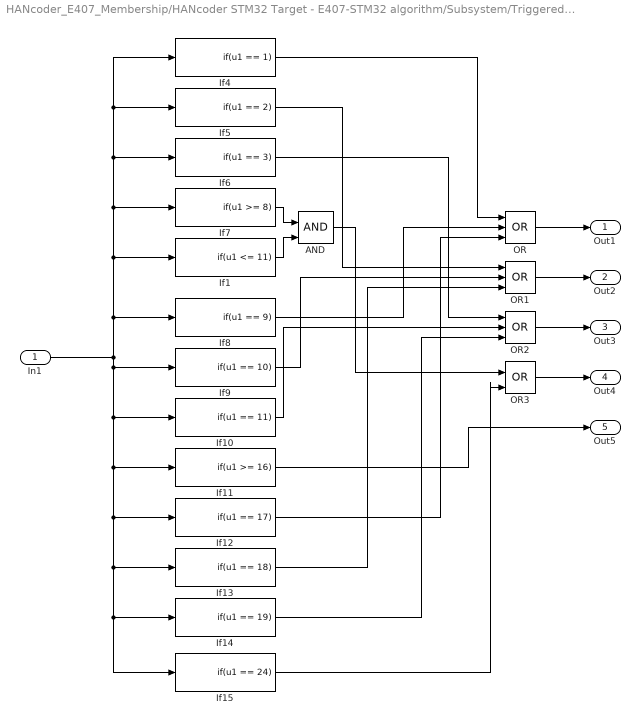
== system HANcoder_E407_Membership/HANcoder STM32 Target - E407-STM32 algorithm/Subsystem/Triggered Subsystem1/Subsystem2 ==
  In1 : Inport
  AND : Logic  IconShape=distinctive  AllPortsSameDT=off  OutDataTypeStr=boolean
  If1 : If  IfExpression=u1 <= 11  ShowElse=off
  If10 : If  IfExpression=u1 == 11  ShowElse=off
  If11 : If  IfExpression=u1 >= 16  ShowElse=off
  If12 : If  IfExpression=u1 == 17  ShowElse=off
  If13 : If  IfExpression=u1 == 18  ShowElse=off
  If14 : If  IfExpression=u1 == 19  ShowElse=off
  If15 : If  IfExpression=u1 == 24  ShowElse=off
  If4 : If  IfExpression=u1 == 1  ShowElse=off
  If5 : If  IfExpression=u1 == 2  ShowElse=off
  If6 : If  IfExpression=u1 == 3  ShowElse=off
  If7 : If  IfExpression=u1 >= 8  ShowElse=off
  If8 : If  IfExpression=u1 == 9  ShowElse=off
  If9 : If  IfExpression=u1 == 10  ShowElse=off
  OR : Logic  Operator=OR  Inputs=3  IconShape=distinctive  AllPortsSameDT=off  OutDataTypeStr=boolean
  OR1 : Logic  Operator=OR  Inputs=3  IconShape=distinctive  AllPortsSameDT=off  OutDataTypeStr=boolean
  OR2 : Logic  Operator=OR  Inputs=3  IconShape=distinctive  AllPortsSameDT=off  OutDataTypeStr=boolean
  OR3 : Logic  Operator=OR  IconShape=distinctive  AllPortsSameDT=off  OutDataTypeStr=boolean
  Out1 : Outport
  Out2 : Outport  Port=2
  Out3 : Outport  Port=3
  Out4 : Outport  Port=4
  Out5 : Outport  Port=5
  wires:
  In1/1 -> If13/1, If14/1, If15/1, If12/1, If11/1, If10/1, If9/1, If1/1, If7/1, If6/1, If5/1, If4/1, If8/1
  OR/1 -> Out1/1
  If4/1 -> OR/1
  If8/1 -> OR/2
  If12/1 -> OR/3
  OR1/1 -> Out2/1
  If5/1 -> OR1/1
  If9/1 -> OR1/2
  If13/1 -> OR1/3
  OR2/1 -> Out3/1
  If6/1 -> OR2/1
  If10/1 -> OR2/2
  If14/1 -> OR2/3
  If15/1 -> OR3/2
  OR3/1 -> Out4/1
  If11/1 -> Out5/1
  If7/1 -> AND/1
  If1/1 -> AND/2
  AND/1 -> OR3/1

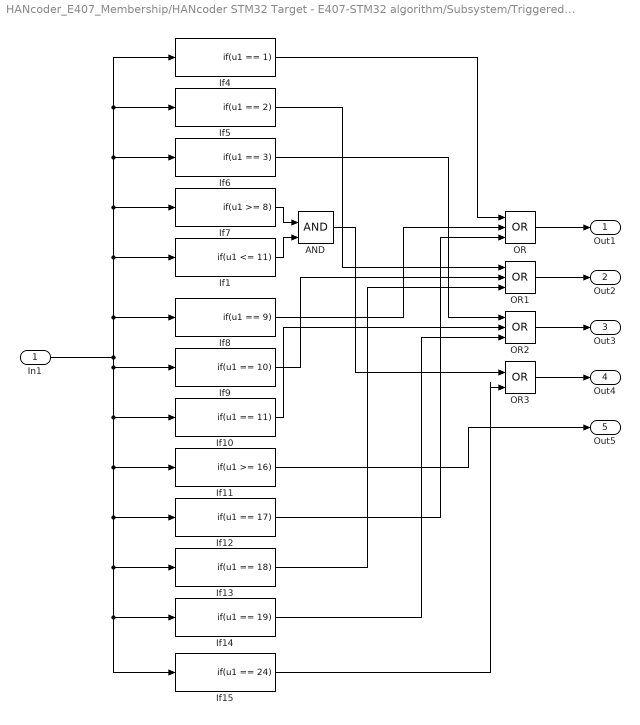
== system HANcoder_E407_Membership/HANcoder STM32 Target - E407-STM32 algorithm/Subsystem/Triggered Subsystem1/Subsystem4 ==
  In1 : Inport
  AND : Logic  IconShape=distinctive  AllPortsSameDT=off  OutDataTypeStr=boolean
  If1 : If  IfExpression=u1 <= 11  ShowElse=off
  If10 : If  IfExpression=u1 == 11  ShowElse=off
  If11 : If  IfExpression=u1 >= 16  ShowElse=off
  If12 : If  IfExpression=u1 == 17  ShowElse=off
  If13 : If  IfExpression=u1 == 18  ShowElse=off
  If14 : If  IfExpression=u1 == 19  ShowElse=off
  If15 : If  IfExpression=u1 == 24  ShowElse=off
  If4 : If  IfExpression=u1 == 1  ShowElse=off
  If5 : If  IfExpression=u1 == 2  ShowElse=off
  If6 : If  IfExpression=u1 == 3  ShowElse=off
  If7 : If  IfExpression=u1 >= 8  ShowElse=off
  If8 : If  IfExpression=u1 == 9  ShowElse=off
  If9 : If  IfExpression=u1 == 10  ShowElse=off
  OR : Logic  Operator=OR  Inputs=3  IconShape=distinctive  AllPortsSameDT=off  OutDataTypeStr=boolean
  OR1 : Logic  Operator=OR  Inputs=3  IconShape=distinctive  AllPortsSameDT=off  OutDataTypeStr=boolean
  OR2 : Logic  Operator=OR  Inputs=3  IconShape=distinctive  AllPortsSameDT=off  OutDataTypeStr=boolean
  OR3 : Logic  Operator=OR  IconShape=distinctive  AllPortsSameDT=off  OutDataTypeStr=boolean
  Out1 : Outport
  Out2 : Outport  Port=2
  Out3 : Outport  Port=3
  Out4 : Outport  Port=4
  Out5 : Outport  Port=5
  wires:
  In1/1 -> If13/1, If14/1, If15/1, If12/1, If11/1, If10/1, If9/1, If1/1, If7/1, If6/1, If5/1, If4/1, If8/1
  OR/1 -> Out1/1
  If4/1 -> OR/1
  If8/1 -> OR/2
  If12/1 -> OR/3
  OR1/1 -> Out2/1
  If5/1 -> OR1/1
  If9/1 -> OR1/2
  If13/1 -> OR1/3
  OR2/1 -> Out3/1
  If6/1 -> OR2/1
  If10/1 -> OR2/2
  If14/1 -> OR2/3
  If15/1 -> OR3/2
  OR3/1 -> Out4/1
  If11/1 -> Out5/1
  If7/1 -> AND/1
  If1/1 -> AND/2
  AND/1 -> OR3/1

== system HANcoder_E407_Membership/HANcoder STM32 Target - E407-STM32 algorithm/Subsystem/Triggered Subsystem/Subsystem/If Action Subsystem ==
  In1 : Inport
  Action Port : ActionPort  ActionPortLabel=if(u1 == 0)
  Out1 : Outport
  wires:
  In1/1 -> Out1/1

== system HANcoder_E407_Membership/HANcoder STM32 Target - E407-STM32 algorithm/Subsystem/Triggered Subsystem/Subsystem/If Action Subsystem1 ==
  In1 : Inport
  Action Port : ActionPort  ActionPortLabel=else
  Gain : Gain  Gain=2
  2 : Outport
  wires:
  In1/1 -> Gain/1
  Gain/1 -> 2/1

== system HANcoder_E407_Membership/HANcoder STM32 Target - E407-STM32 algorithm/Subsystem/Triggered Subsystem/Subsystem/If Action Subsystem2 ==
  In1 : Inport
  Action Port : ActionPort  ActionPortLabel=if(u1 == 0)
  Out1 : Outport
  wires:
  In1/1 -> Out1/1

== system HANcoder_E407_Membership/HANcoder STM32 Target - E407-STM32 algorithm/Subsystem/Triggered Subsystem/Subsystem/If Action Subsystem3 ==
  In1 : Inport
  Action Port : ActionPort  ActionPortLabel=else
  Gain : Gain  Gain=2
  2 : Outport
  wires:
  In1/1 -> Gain/1
  Gain/1 -> 2/1
